simulink library "DAEMOT_Lib"  (R2019b)
settings: Solver=ode45  StartTime=0.0  StopTime=10.0  FixedStep=0.1  RelTol=1e-3
undefined symbols (not defined in the file or in its folder): Controller, CP, Ctrl, Ctrl_Fcn, Elec1, f, F2, Fluid, lag1, Mission, Moody, PropellerProp, rev_comms_sink
libraries: $bdroot x200, instrumentlib x21, simulink x5, dspsigops x2
(part 11 of 13)

== system DAEMOT_Lib/Electrical/Battery/Property ==
  I : Inport
  T_m : Inport  Port=2
  SOC : Inport  Port=3
  " " : Lookup  InputValues=cell.Ent_SOC  Table=cell.dUdt
  " " : Lookup  InputValues=cell.V_SOC  Table=cell.Vocv  LookUpMeth=Interpolation-Use End Values
  Fcn{1..5} (5 alike) : Fcn  Expr=((u(1)-u(3))/(1+exp(-50*u(2))))+u(3)
  Gain : Gain  Gain=Ns
  Mux : Mux  Inputs=7
  Mux{1..5} (5 alike) : Mux  Inputs=3
  n-D Lookup Table1 : Lookup_n-D  BreakpointsForDimension1=cell.RC_SOC_c  BreakpointsForDimension2=cell.Temp  BreakpointsForDimension3=[5, 7]  Table=cell.Rs_c  RndMeth=Simplest  InputSameDT=on
  n-D Lookup Table13 : Lookup_n-D  BreakpointsForDimension1=cell.RC_SOC_d  BreakpointsForDimension2=cell.Temp  BreakpointsForDimension3=[5, 7]  Table=cell.Rs_d  RndMeth=Simplest  InputSameDT=on
  n-D Lookup Table2 : Lookup_n-D  BreakpointsForDimension1=cell.RC_SOC_d  BreakpointsForDimension2=cell.Temp  BreakpointsForDimension3=[5, 7]  Table=cell.R1_d  RndMeth=Simplest  InputSameDT=on
  n-D Lookup Table3 : Lookup_n-D  BreakpointsForDimension1=cell.RC_SOC_c  BreakpointsForDimension2=cell.Temp  BreakpointsForDimension3=[5, 7]  Table=cell.R1_c  RndMeth=Simplest  InputSameDT=on
  n-D Lookup Table4 : Lookup_n-D  BreakpointsForDimension1=cell.RC_SOC_d  BreakpointsForDimension2=cell.Temp  BreakpointsForDimension3=[5, 7]  Table=cell.C1_d  RndMeth=Simplest  InputSameDT=on
  n-D Lookup Table5 : Lookup_n-D  BreakpointsForDimension1=cell.RC_SOC_c  BreakpointsForDimension2=cell.Temp  BreakpointsForDimension3=[5, 7]  Table=cell.C1_c  RndMeth=Simplest  InputSameDT=on
  n-D Lookup Table6 : Lookup_n-D  BreakpointsForDimension1=cell.RC_SOC_d  BreakpointsForDimension2=cell.Temp  BreakpointsForDimension3=[5, 7]  Table=cell.R2_d  RndMeth=Simplest  InputSameDT=on
  n-D Lookup Table7 : Lookup_n-D  BreakpointsForDimension1=cell.RC_SOC_c  BreakpointsForDimension2=cell.Temp  BreakpointsForDimension3=[5, 7]  Table=cell.R2_c  RndMeth=Simplest  InputSameDT=on
  n-D Lookup Table8 : Lookup_n-D  BreakpointsForDimension1=cell.RC_SOC_d  BreakpointsForDimension2=cell.Temp  BreakpointsForDimension3=[5, 7]  Table=cell.C2_d  RndMeth=Simplest  InputSameDT=on
  n-D Lookup Table9 : Lookup_n-D  BreakpointsForDimension1=cell.RC_SOC_c  BreakpointsForDimension2=cell.Temp  BreakpointsForDimension3=[5, 7]  Table=cell.C2_c  RndMeth=Simplest  InputSameDT=on
  Props : Outport
  wires:
  Gain/1 -> Mux/7
  Mux/1 -> Props/1
  " "/1 -> Gain/1  "V_ocv"
  " "/1 -> Mux/6  "dU_dt"
  Fcn1/1 -> Mux/1  "Rs"
  T_m/1 -> n-D Lookup Table9/2, n-D Lookup Table8/2, n-D Lookup Table7/2, n-D Lookup Table6/2, n-D Lookup Table5/2, n-D Lookup Table4/2, n-D Lookup Table3/2, n-D Lookup Table2/2, n-D Lookup Table1/2, n-D Lookup Table13/2
  SOC/1 -> n-D Lookup Table9/1, " "/1, " "/1, n-D Lookup Table8/1, n-D Lookup Table7/1, n-D Lookup Table6/1, n-D Lookup Table5/1, n-D Lookup Table4/1, n-D Lookup Table3/1, n-D Lookup Table2/1, n-D Lookup Table1/1, n-D Lookup Table13/1
  I/1 -> Mux2/2, Mux1/2, Mux5/2, Mux4/2, Mux3/2
  Fcn5/1 -> Mux/5  "C2"
  Fcn4/1 -> Mux/4  "R2"
  Fcn2/1 -> Mux/2  "R1"
  Fcn3/1 -> Mux/3  "C1"
  Mux2/1 -> Fcn1/1
  n-D Lookup Table1/1 -> Mux2/3
  n-D Lookup Table13/1 -> Mux2/1
  Mux1/1 -> Fcn2/1
  n-D Lookup Table2/1 -> Mux1/1
  n-D Lookup Table3/1 -> Mux1/3
  Mux3/1 -> Fcn3/1
  n-D Lookup Table4/1 -> Mux3/1
  n-D Lookup Table5/1 -> Mux3/3
  Mux4/1 -> Fcn4/1
  n-D Lookup Table6/1 -> Mux4/1
  n-D Lookup Table7/1 -> Mux4/3
  Mux5/1 -> Fcn5/1
  n-D Lookup Table8/1 -> Mux5/1
  n-D Lookup Table9/1 -> Mux5/3

== system DAEMOT_Lib/Electrical/Battery/Sink1 ==
  In1 : Inport
  tag scope: gdata_DAEMOT_LibElectricalBatterySink1=global
  wires:
  In1/1 -> [gdata_DAEMOT_LibElectricalBatterySink1]

== system DAEMOT_Lib/Electrical/Battery/Source1 ==
  Out1 : Outport
  wires:
  [NULL] -> Out1/1

== system DAEMOT_Lib/Electrical/Battery/Source2 ==
  Out1 : Outport
  wires:
  [NULL] -> Out1/1

== system DAEMOT_Lib/Electrical/Current Sink/Sink1 ==
  In1 : Inport
  tag scope: gdata_DAEMOT_LibElectricalCurrentSinkSink1=global
  wires:
  In1/1 -> [gdata_DAEMOT_LibElectricalCurrentSinkSink1]

== system DAEMOT_Lib/Electrical/Current Source/Source1 ==
  Out1 : Outport  VectorParamsAs1DForOutWhenUnconnected=off
  wires:
  [NULL] -> Out1/1

== system DAEMOT_Lib/Electrical/ESC/Data_Sink ==
  " " : Inport
  tag scope: gdata_ElectricalESCData_Sink=global
  wires:
  " "/1 -> [gdata_ElectricalESCData_Sink]

== system DAEMOT_Lib/Electrical/ESC/Sink1 ==
  In1 : Inport
  tag scope: gdata_DAEMOT_LibElectricalESCSink1=global
  wires:
  In1/1 -> [gdata_DAEMOT_LibElectricalESCSink1]

== system DAEMOT_Lib/Electrical/Effort Sink/Sink1 ==
  In1 : Inport
  tag scope: gdata_DAEMOT_LibElectricalEffortSinkSink1=global
  wires:
  In1/1 -> [gdata_DAEMOT_LibElectricalEffortSinkSink1]

== system DAEMOT_Lib/Electrical/Effort Source/Source1 ==
  Out1 : Outport  VectorParamsAs1DForOutWhenUnconnected=off
  wires:
  [NULL] -> Out1/1

== system DAEMOT_Lib/Electrical/Engine/Data_Sink ==
  " " : Inport
  tag scope: gdata_ElectricalEngineData_Sink=global
  wires:
  " "/1 -> [gdata_ElectricalEngineData_Sink]

== system DAEMOT_Lib/Electrical/Engine/Dynamic Saturation ==
  up : Inport
  u : Inport  Port=2
  dn : Inport  Port=3
  LowerRelop1 : RelationalOperator  DisableCoverage=on  Operator=>  OutDataTypeStr=boolean  ZeroCross=off  RndMeth=Nearest
  Switch : Switch  Criteria=u2 ~= 0  OutDataTypeStr=Inherit: Inherit via back propagation  ZeroCross=off
  Switch2 : Switch  Criteria=u2 ~= 0  OutMin=0  OutMax=1  OutDataTypeStr=Inherit: Inherit via back propagation  ZeroCross=off
  UpperRelop : RelationalOperator  DisableCoverage=on  Operator=<  OutDataTypeStr=boolean  ZeroCross=off  RndMeth=Nearest
  Out1 : Outport
  wires:
  Switch2/1 -> Out1/1
  up/1 -> Switch2/1, LowerRelop1/2
  UpperRelop/1 -> Switch/2
  dn/1 -> UpperRelop/2, Switch/1
  LowerRelop1/1 -> Switch2/2
  Switch/1 -> Switch2/3
  u/1 -> UpperRelop/1, Switch/3, LowerRelop1/1

== system DAEMOT_Lib/Electrical/Engine/Sink1 ==
  In1 : Inport
  tag scope: gdata_DAEMOT_LibElectricalEngineSink1=global
  wires:
  In1/1 -> [gdata_DAEMOT_LibElectricalEngineSink1]

== system DAEMOT_Lib/Electrical/Gearbox/Data_Sink ==
  " " : Inport
  tag scope: gdata_ElectricalGearboxData_Sink=global
  wires:
  " "/1 -> [gdata_ElectricalGearboxData_Sink]

== system DAEMOT_Lib/Electrical/Gearbox/Sink1 ==
  In1 : Inport
  tag scope: gdata_DAEMOT_LibElectricalGearboxSink1=global
  wires:
  In1/1 -> [gdata_DAEMOT_LibElectricalGearboxSink1]

== system DAEMOT_Lib/Electrical/Gearbox/Source1 ==
  Out1 : Outport
  wires:
  [NULL] -> Out1/1

== system DAEMOT_Lib/Electrical/Inverter/Data_Sink ==
  " " : Inport
  tag scope: gdata_ElectricalInverterData_Sink=global
  wires:
  " "/1 -> [gdata_ElectricalInverterData_Sink]

== system DAEMOT_Lib/Electrical/Inverter/Sink1 ==
  In1 : Inport
  tag scope: gdata_DAEMOT_LibElectricalInverterSink1=global
  wires:
  In1/1 -> [gdata_DAEMOT_LibElectricalInverterSink1]

== system DAEMOT_Lib/Electrical/Inverter/Source1 ==
  Out1 : Outport
  wires:
  [NULL] -> Out1/1

== system DAEMOT_Lib/Electrical/Inverter/Source2 ==
  Out1 : Outport
  wires:
  [NULL] -> Out1/1

== system DAEMOT_Lib/Electrical/Motor/Data_Sink ==
  " " : Inport
  tag scope: gdata_ElectricalMotorData_Sink=global
  wires:
  " "/1 -> [gdata_ElectricalMotorData_Sink]

== system DAEMOT_Lib/Electrical/Motor/Sink1 ==
  In1 : Inport
  tag scope: gdata_DAEMOT_LibElectricalMotorSink1=global
  wires:
  In1/1 -> [gdata_DAEMOT_LibElectricalMotorSink1]

== system DAEMOT_Lib/Electrical/Motor/Source1 ==
  Out1 : Outport
  wires:
  [NULL] -> Out1/1

== system DAEMOT_Lib/Electrical/Motor/Source2 ==
  Out1 : Outport
  wires:
  [NULL] -> Out1/1

== system DAEMOT_Lib/Electrical/MotorNoShaft/Data_Sink ==
  " " : Inport
  tag scope: gdata_ElectricalMotorNoShaftData_Sink=global
  wires:
  " "/1 -> [gdata_ElectricalMotorNoShaftData_Sink]

== system DAEMOT_Lib/Electrical/MotorNoShaft/Sink1 ==
  In1 : Inport
  tag scope: gdata_DAEMOT_LibElectricalMotorNoShaftSink1=global
  wires:
  In1/1 -> [gdata_DAEMOT_LibElectricalMotorNoShaftSink1]

== system DAEMOT_Lib/Electrical/MotorNoShaft/Source1 ==
  Out1 : Outport
  wires:
  [NULL] -> Out1/1

== system DAEMOT_Lib/Electrical/MotorNoShaft/Source2 ==
  Out1 : Outport
  wires:
  [NULL] -> Out1/1

== system DAEMOT_Lib/Electrical/Shaft/Data_Sink ==
  " " : Inport
  tag scope: gdata_ElectricalShaftData_Sink=global
  wires:
  " "/1 -> [gdata_ElectricalShaftData_Sink]

== system DAEMOT_Lib/Electrical/Shaft/Sink1 ==
  In1 : Inport
  tag scope: gdata_DAEMOT_LibElectricalShaftSink1=global
  wires:
  In1/1 -> [gdata_DAEMOT_LibElectricalShaftSink1]

== system DAEMOT_Lib/Electrical/Shaft/Source1 ==
  Out1 : Outport
  wires:
  [NULL] -> Out1/1

== system DAEMOT_Lib/Electrical/Speed Source/Source1 ==
  Out1 : Outport  VectorParamsAs1DForOutWhenUnconnected=off
  wires:
  [NULL] -> Out1/1

== system DAEMOT_Lib/Electrical/Torque Sink/Sink1 ==
  In1 : Inport
  tag scope: gdata_DAEMOT_LibElectricalTorqueSinkSink1=global
  wires:
  In1/1 -> [gdata_DAEMOT_LibElectricalTorqueSinkSink1]

== system DAEMOT_Lib/Electrical/UAV/Property ==
  v : Inport
  w : Inport  Port=2
  " C_L" : Lookup  InputValues=PropellerProp.J  Table=PropellerProp.C_L
  " C_T" : Lookup  InputValues=PropellerProp.J  Table=PropellerProp.C_T
  " eta" : Lookup  InputValues=PropellerProp.J  Table=PropellerProp.eta
  Divide : Product  Inputs=*/
  Gain : Gain  Gain=2*pi
  Gain1 : Gain  Gain=d
  Mux : Mux
  Scope : Scope
  Props : Outport  VectorParamsAs1DForOutWhenUnconnected=off
  wires:
  Mux/1 -> Props/1
  w/1 -> Gain1/1
  v/1 -> Gain/1
  Gain/1 -> Divide/1
  Gain1/1 -> Divide/2
  Divide/1 -> " eta"/1, " C_L"/1, " C_T"/1, Scope/1, Mux/1  "J"
  " C_T"/1 -> Mux/2  "C_T"
  " C_L"/1 -> Mux/3  "C_L"
  " eta"/1 -> Mux/4  "eta"

== system DAEMOT_Lib/Electrical/Ultracapacitor/Props ==
  Constant : Constant  Value=R_i
  Constant1 : Constant  Value=C_i0
  Constant2 : Constant  Value=C_i1
  Constant3 : Constant  Value=R_d
  Constant4 : Constant  Value=C_d
  Constant5 : Constant  Value=R_l
  Constant6 : Constant  Value=C_l
  Constant7 : Constant  Value=R_leak
  Mux : Mux  Inputs=8
  props : Outport  VectorParamsAs1DForOutWhenUnconnected=off
  wires:
  Constant/1 -> Mux/1
  Constant1/1 -> Mux/2
  Mux/1 -> props/1
  Constant2/1 -> Mux/3
  Constant3/1 -> Mux/4
  Constant4/1 -> Mux/5
  Constant5/1 -> Mux/6
  Constant6/1 -> Mux/7
  Constant7/1 -> Mux/8

== system DAEMOT_Lib/Electrical/Ultracapacitor/Sink1 ==
  In1 : Inport
  Scope : Scope
  tag scope: gdata_DAEMOT_LibElectricalUltracapacitorSink1=global
  wires:
  In1/1 -> Scope/1, [gdata_DAEMOT_LibElectricalUltracapacitorSink1]

== system DAEMOT_Lib/Electrical/Voltage Sink/Sink1 ==
  In1 : Inport
  tag scope: gdata_DAEMOT_LibElectricalVoltageSinkSink1=global
  wires:
  In1/1 -> [gdata_DAEMOT_LibElectricalVoltageSinkSink1]

== system DAEMOT_Lib/Electrical/Voltage Source/Source1 ==
  Out1 : Outport  VectorParamsAs1DForOutWhenUnconnected=off
  wires:
  [NULL] -> Out1/1

== system DAEMOT_Lib/Electrical/wye2del/Data_Sink ==
  " " : Inport
  tag scope: gdata_Electricalwye2delData_Sink=global
  wires:
  " "/1 -> [gdata_Electricalwye2delData_Sink]

== system DAEMOT_Lib/Electrical/wye2del/Sink1 ==
  In1 : Inport
  tag scope: gdata_DAEMOT_LibElectricalwye2delSink1=global
  wires:
  In1/1 -> [gdata_DAEMOT_LibElectricalwye2delSink1]

== system DAEMOT_Lib/Electrical/wye2del/Source1 ==
  Out1 : Outport
  wires:
  [NULL] -> Out1/1

== system DAEMOT_Lib/Legacy Components/Fan1/Sink1 ==
  In1 : Inport
  tag scope: gdata_DAEMOT_LibLegacyComponentsFan1Sink1=global
  wires:
  In1/1 -> [gdata_DAEMOT_LibLegacyComponentsFan1Sink1]

== system DAEMOT_Lib/Legacy Components/Flow Flow Source (Pressure)/Source1 ==
  Out1 : Outport  VectorParamsAs1DForOutWhenUnconnected=off
  wires:
  [gdata_Thermal_System_BUSM2FSink2] -> Out1/1

== system DAEMOT_Lib/Legacy Components/Flow Source (Mass Flow Rate)/Source1 ==
  Out1 : Outport  VectorParamsAs1DForOutWhenUnconnected=off
  wires:
  [gdata_Thermal_System_BUSM2FSink2] -> Out1/1

== system DAEMOT_Lib/Legacy Components/Flow Split_Junction_Wall/Source1 ==
  Out1 : Outport  VectorParamsAs1DForOutWhenUnconnected=off
  wires:
  [NULL] -> Out1/1

== system DAEMOT_Lib/Legacy Components/Graph Sink/Sink1 ==
  In1 : Inport
  tag scope: gdata_DAEMOT_LibLegacyComponentsGraphSinkSink1=global
  wires:
  In1/1 -> [gdata_DAEMOT_LibLegacyComponentsGraphSinkSink1]

== system DAEMOT_Lib/Legacy Components/Graph Source/Source1 ==
  Out1 : Outport  VectorParamsAs1DForOutWhenUnconnected=off
  wires:
  [NULL] -> Out1/1

== system DAEMOT_Lib/Legacy Components/Heat Sink (Temp)/Sink1 ==
  In1 : Inport
  tag scope: gdata_DAEMOT_LibLegacyComponentsHeatSinkTempSink1=global
  wires:
  In1/1 -> [gdata_DAEMOT_LibLegacyComponentsHeatSinkTempSink1]

== system DAEMOT_Lib/Legacy Components/Pipe_M_to_M/Props ==
  P : Inport
  T : Inport  Port=2
  Divide : Product  Inputs=*/
  Fcn : Fcn  Expr=0.99*u
  Subtract : Sum  Inputs=+-
  Subtract1 : Sum  Inputs=+-
  n-D Lookup Table1 : Lookup_n-D  BreakpointsForDimension1=Fluid.P  BreakpointsForDimension2=Fluid.T  BreakpointsForDimension3=[5, 7]  Table=Fluid.Rho_pt  ExtrapMethod=Clip  UseLastTableValue=on  RndMeth=Simplest  InputSameDT=on
  n-D Lookup Table5 : Lookup_n-D  BreakpointsForDimension1=Fluid.P  BreakpointsForDimension2=Fluid.T  BreakpointsForDimension3=[5, 7]  Table=Fluid.Rho_pt  ExtrapMethod=Clip  UseLastTableValue=on  RndMeth=Simplest  InputSameDT=on
  Rho : Outport  VectorParamsAs1DForOutWhenUnconnected=off
  dRho_dP : Outport  Port=2  VectorParamsAs1DForOutWhenUnconnected=off
  wires:
  T/1 -> n-D Lookup Table5/2, n-D Lookup Table1/2
  n-D Lookup Table5/1 -> Subtract/1, Rho/1
  P/1 -> Subtract1/1, Fcn/1, n-D Lookup Table5/1
  Fcn/1 -> n-D Lookup Table1/1, Subtract1/2
  n-D Lookup Table1/1 -> Subtract/2
  Subtract/1 -> Divide/1
  Subtract1/1 -> Divide/2
  Divide/1 -> dRho_dP/1

== system DAEMOT_Lib/Legacy Components/Power Sink (Current)/Sink1 ==
  In1 : Inport
  tag scope: gdata_DAEMOT_LibLegacyComponentsPowerSinkCurrentSink1=global
  wires:
  In1/1 -> [gdata_DAEMOT_LibLegacyComponentsPowerSinkCurrentSink1]

== system DAEMOT_Lib/Legacy Components/Power Source (Voltage)/Source1 ==
  Out1 : Outport  VectorParamsAs1DForOutWhenUnconnected=off
  wires:
  [NULL] -> Out1/1

== system DAEMOT_Lib/Legacy Components/Static Flow Split/Sink1 ==
  In1 : Inport
  tag scope: gdata_DAEMOT_LibLegacyComponentsStaticFlowSplitSink1=global
  wires:
  In1/1 -> [gdata_DAEMOT_LibLegacyComponentsStaticFlowSplitSink1]

== system DAEMOT_Lib/Legacy Components/Static Flow Split/Source1 ==
  Out1 : Outport  VectorParamsAs1DForOutWhenUnconnected=off
  wires:
  [gdata_Thermal_System_BUSFuelPumSink1] -> Out1/1

== system DAEMOT_Lib/Legacy Components/UDP_Controller_SR_old/From Controller ==
  MEASUREMENTS1 : Subsystem  mask{n_meas=out_size}
      mask prompts: n_meas "Number of measurements from LabView"
      mask init:
      | h = gcbh;
      | param = get(h);
      | blk = [param.Path, '/', param.Name,'/UDP Receive'];
      | h = get_param(blk,'handle');
      | 
      | set_param(h,'DataSize',['[',num2str(n_meas),' 1]'])
      mask Display:
      | if n_meas > 1
      |     port_label('output',1,['Mux - ',num2str(n_meas),' signals'])
      | else
      |     port_label('output',1,['Mux - ',num2str(n_meas),' signal'])
      | end
  Out1 : Outport  VectorParamsAs1DForOutWhenUnconnected=off
  wires:
  MEASUREMENTS1/1(Out) -> Out1/1

== system DAEMOT_Lib/Legacy Components/UDP_Controller_SR_old/To Controller ==
  " " : Inport
  UDP Send : instrumentlib/UDP Send  Host=localhost  Port=61176  LocalPort=61177  EnablePortSharing=off  ByteOrder=BigEndian  OutputDatagramPacketSize=512  EnableBlockingMode=on  LocalAddress=0.0.0.0
      settings: SourceProductName=Instrument Control Toolbox
  wires:
  " "/1 -> UDP Send/1

== system DAEMOT_Lib/Legacy Components/UDP_Controller_old/From Controller ==
  " " : Inport
  UDP Send : instrumentlib/UDP Send  Host=localhost  Port=61167  LocalPort=61166  EnablePortSharing=off  ByteOrder=BigEndian  OutputDatagramPacketSize=512  EnableBlockingMode=on  LocalAddress=0.0.0.0
      settings: SourceProductName=Instrument Control Toolbox
  Zero-Order Hold : ZeroOrderHold  Commented=through  SampleTime=0.1
  wires:
  " "/1 -> Zero-Order Hold/1
  Zero-Order Hold/1 -> UDP Send/1

== system DAEMOT_Lib/Legacy Components/UDP_Controller_old/To Controller ==
  UDP Receive : instrumentlib/UDP Receive  Host=localhost  Port=61177  LocalPort=61176  EnablePortSharing=off  GetLatestData=off  DataSize=[1 1]  DataType=double  ASCIIFormatting=%f,  Terminator=LF  ByteOrder=BigEndian  EnableBlockingMode=on  Timeout=6  SampleTime=1  LocalAddress=0.0.0.0
      settings: SourceProductName=Instrument Control Toolbox
  Out : Outport  VectorParamsAs1DForOutWhenUnconnected=off
  wires:
  UDP Receive/1 -> Out/1

== system DAEMOT_Lib/Legacy Components/Upper to Lower Edge Preview_old/Mission Preview1 ==
  Trajectory : Inport
  Time : Inport  Port=2
  Add : Sum
  Bias : Bias  Bias=+dt_l*linspace(0,(hor_l-1),hor_l)
  Constant : Constant  Value=0:dt_l:((hor_u)*dt_u-1)  VectorParams1D=off
  Digital Clock : DigitalClock  SampleTime=dt_l
  Display{,1..3} (4 alike) : Display
  Lookup Table Dynamic : simulink/Lookup Tables/Lookup Table Dynamic  LookUpMeth=Use Input Below  OutDataType=fixdt('double')  OutScaling=[]  OutputDataTypeScalingMode=Specify via dialog  OutDataTypeStr=double  DoSatur=off
      settings: SourceProductName=Simulink
  MATLAB Function : MATLAB Function  Commented=on  TreatAsAtomicUnit=on
  MATLAB Function1 : MATLAB Function  TreatAsAtomicUnit=on
  Reshape : Reshape  OutputDimensionality=Row vector (2-D)
  Reshape1 : Reshape
  References : Outport  VectorParamsAs1DForOutWhenUnconnected=off
  wires:
  Reshape/1 -> References/1, Display3/1
  MATLAB Function1/1(y) -> Lookup Table Dynamic/3, Display2/1
  Reshape1/1 -> MATLAB Function1/1(u)
  Constant/1 -> Add/2
  Time/1 -> Add/1
  Add/1 -> Lookup Table Dynamic/2, Display1/1
  Trajectory/1 -> Reshape1/1
  Lookup Table Dynamic/1 -> Reshape/1
  Bias/1 -> Lookup Table Dynamic/1, Display/1
  Digital Clock/1 -> Bias/1

== system DAEMOT_Lib/Support Functions/Generic Graph Model/Variant Subsystem ==
  Inputs : Inport
  Source Vertex : Inport  Port=2
  Source Edge : Inport  Port=3
  DAE Graph : Subsystem  VariantControl=DAE_Graph
  Dynamic Graph : Subsystem  VariantControl=Dynamic_Graph
  States : Outport
  Power Flows : Outport  Port=2

== system DAEMOT_Lib/Support Functions/Generic Sink/Sink1 ==
  In1 : Inport
  tag scope: gdata_DAEMOT_LibSupportFunctionsGenericSinkSink1=global
  wires:
  In1/1 -> [gdata_DAEMOT_LibSupportFunctionsGenericSinkSink1]

== system DAEMOT_Lib/Support Functions/Generic Source/Source1 ==
  Out1 : Outport  VectorParamsAs1DForOutWhenUnconnected=off
  wires:
  [NULL] -> Out1/1

== system DAEMOT_Lib/Support Functions/Real-Time Communication/LabVIEW_UDP ==
  " " : Inport
  Bus Creator : BusCreator  Inputs=15
  Bus Selector : BusSelector  OutputSignals=SimulinkTime,MCM_EnablePropESC,MCM_RPMCommand,MCM_EnableBattCharge,MCM_EnableSGESC,MCM_EnableICE,MCM_GenIMax,MCM_BattIMax,Dyno_Enable,Dyno_C0,Dyno_C1,Dyno_C2,DCDC_Enable0,DCDC_Enable1,DCDC_Enable2,DCDC_Voltage0,DCDC_Voltage1,DCDC_Voltage2,DCDC_Current0,DCDC_Current1,DCDC_Current2,ELoad_voltage_limit_enabled,ELoad_voltage_limit  OutputAsBus=on
  Bus to Vector : BusToVector
  Check_NaN1 : Subsystem  mask{N=n_in}
      mask prompts: N "Number of Signals"
  Demux : Demux  Outputs=15
  UDP Receive : instrumentlib/UDP Receive  Host=localhost  Port=61556  LocalPort=61557  EnablePortSharing=off  GetLatestData=off  DataSize=[15 1]  DataType=double  ASCIIFormatting=%f,  Terminator=LF  ByteOrder=BigEndian  EnableBlockingMode=on  Timeout=10  SampleTime=0.1  LocalAddress=0.0.0.0
      settings: SourceProductName=Instrument Control Toolbox
  UDP Send : instrumentlib/UDP Send  Host=localhost  Port=61556  LocalPort=61557  EnablePortSharing=off  ByteOrder=BigEndian  OutputDatagramPacketSize=512  EnableBlockingMode=on  LocalAddress=0.0.0.0
      settings: SourceProductName=Instrument Control Toolbox
  Zero-Order Hold : ZeroOrderHold  SampleTime=0.1
  Out : Outport  VectorParamsAs1DForOutWhenUnconnected=off
  wires:
  Bus to Vector/1 -> Zero-Order Hold/1
  Bus Selector/1 -> Bus to Vector/1
  Zero-Order Hold/1 -> UDP Send/1
  " "/1 -> Bus Selector/1
  Bus Creator/1 -> Out/1
  UDP Receive/1 -> Check_NaN1/1(In1)
  Check_NaN1/1(Out1) -> Demux/1
  Demux/1 -> Bus Creator/1  "Test Time"
  Demux/2 -> Bus Creator/2  "PackVoltage"
  Demux/3 -> Bus Creator/3  "(MCM) Bus Voltage [V]"
  Demux/4 -> Bus Creator/4  "(DCDC) Bus Voltage [V]"
  Demux/5 -> Bus Creator/5  "Shunt_SystemBatt"
  Demux/6 -> Bus Creator/6  "(MCM) Bus DC Current [A]"
  Demux/7 -> Bus Creator/7  "Shunt_VoltageSteps"
  Demux/8 -> Bus Creator/8  "(DCDC) Bus DC Current [A]"
  Demux/9 -> Bus Creator/9  "(MCM) Prop DC Current [A]"
  Demux/10 -> Bus Creator/10  "(MCM) Prop Speed [RPM]"
  Demux/11 -> Bus Creator/11  "(MCM) SG DC Current [A]"
  Demux/12 -> Bus Creator/12  "ELoad_voltage_measured"
  Demux/13 -> Bus Creator/13  "ELoad_current_measured"
  Demux/14 -> Bus Creator/14  "Shunt_Channel_A_Load"
  Demux/15 -> Bus Creator/15  "(DCDC) Duty Cycle A"

== system DAEMOT_Lib/Support Functions/Real-Time Communication/UDP_Controller ==
  note: the zero order hold should be unnecessary
      | because everything here has a Ctrl.dt update
      | rate. When operating with Parallel simulations,
      | this block will start in sync with the main simulation.
      | Once the controller calls, the main and parallel sims
      | will operate asynchronously. Upon controller call completion,
      | data is immediately sent to the main sim. The main sim will receive
      | that data at it's update rate (likely 10Hz). At this point, the main sim
      | is ahead of the parallel sim by the time it took to call
      | the controller rounded up to the nearest .1s (assuming
      | 10Hz). However, the parallel sim can now immediately forward
      | simulate to the next UDP recieve and wait for data (The
      | parallel sim is ahead of the main sim for this period). Once the
      | main sim catches up in time, data is sent to and recieved by the
      | parallel sim and the process repeats.
  Controller : Subsystem  TreatAsAtomicUnit=on  SystemSampleTime=0.1
  Display : Display
  Display1 : Display
  From Controller : Subsystem  Priority=3  TreatAsAtomicUnit=on  SystemSampleTime=0.1
  Reshape1 : Reshape  OutputDimensionality=Column vector (2-D)
  Scope : Scope
  Scope1 : Scope
  UDP Receive : instrumentlib/UDP Receive  Priority=2  Host=localhost  Port=61177  LocalPort=61176  EnablePortSharing=off  GetLatestData=off  DataSize=[10 1]  DataType=double  ASCIIFormatting=%f,  Terminator=LF  ByteOrder=BigEndian  EnableBlockingMode=on  Timeout=5.1  SampleTime=0.1  LocalAddress=0.0.0.0
      settings: SourceProductName=Instrument Control Toolbox
  Zero-Order Hold : ZeroOrderHold  Commented=through  SampleTime=Ctrl.dt
  wires:
  Reshape1/1 -> Controller/1(In1), Scope/1
  UDP Receive/1 -> Reshape1/1
  Controller/1(Out1) -> Display/1, Zero-Order Hold/1
  Zero-Order Hold/1 -> Display1/1, From Controller/1(" "), Scope1/1

== system DAEMOT_Lib/Support Functions/Real-Time Communication/UDP_Controller_Debug ==
  Controller : MATLABFcn  MATLABFcn=Controller(u)  OutputDimensions=10
  From Controller : Subsystem  Priority=3  TreatAsAtomicUnit=on  SystemSampleTime=0.1
  Reshape1 : Reshape  OutputDimensionality=Column vector (2-D)
  Scope : Scope
  Scope1 : Scope
  UDP Receive : instrumentlib/UDP Receive  Priority=2  Host=localhost  Port=61177  LocalPort=61176  EnablePortSharing=off  GetLatestData=off  DataSize=[10 1]  DataType=double  ASCIIFormatting=%f,  Terminator=LF  ByteOrder=BigEndian  EnableBlockingMode=on  Timeout=5.1  SampleTime=0.1  LocalAddress=0.0.0.0
      settings: SourceProductName=Instrument Control Toolbox
  wires:
  Controller/1 -> From Controller/1(" "), Scope1/1
  Reshape1/1 -> Scope/1, Controller/1
  UDP Receive/1 -> Reshape1/1

== system DAEMOT_Lib/Support Functions/Real-Time Communication/UDP_Controller_Recieve ==
  Bus Creator : BusCreator  Inputs=2
  From Controller : Subsystem  Commented=on  TreatAsAtomicUnit=on  SystemSampleTime=.1
  Reshape : Reshape
  Sample and Hold : dspsigops/Sample and Hold  trig=Rising edge  initCond=Initial  latchinput=off
  TCP/IP Receive : instrumentlib/TCP//IP Receive  Priority=2  Commented=on  Host=localhost  Port=50000  DataSize=[1 1]  EnableBlockingMode=on  Timeout=3  SampleTime=.1  DataType=double  ByteOrder=BigEndian  ASCIIFormatting=%f,  Terminator=LF
      settings: SourceProductName=Instrument Control Toolbox
  UDP Receive : instrumentlib/UDP Receive  Priority=3  Host=localhost  Port=61166  LocalPort=61167  EnablePortSharing=off  GetLatestData=off  DataSize=[10 1]  DataType=double  ASCIIFormatting=%f,  Terminator=LF  ByteOrder=BigEndian  EnableBlockingMode=off  Timeout=10  SampleTime=0.1  LocalAddress=0.0.0.0
      settings: SourceProductName=Instrument Control Toolbox
  Zero-Order Hold : ZeroOrderHold  SampleTime=0.1
  Output : Outport  VectorParamsAs1DForOutWhenUnconnected=off
  wires:
  Bus Creator/1 -> Output/1
  Zero-Order Hold/1 -> Bus Creator/2  "Output at Update"
  Sample and Hold/1 -> Zero-Order Hold/1, Bus Creator/1  "Immediate Output"
  UDP Receive/2 -> Sample and Hold/Trigger
  UDP Receive/1 -> Reshape/1  "Recieved"
  Reshape/1 -> Sample and Hold/1

== system DAEMOT_Lib/Support Functions/Real-Time Communication/UDP_Controller_Recieve_Debug ==
  Reshape : Reshape
  Scope : Scope
  UDP Receive : instrumentlib/UDP Receive  Priority=3  Host=localhost  Port=61166  LocalPort=61167  EnablePortSharing=off  GetLatestData=off  DataSize=[10 1]  DataType=double  ASCIIFormatting=%f,  Terminator=LF  ByteOrder=BigEndian  EnableBlockingMode=on  Timeout=10  SampleTime=0.1  LocalAddress=0.0.0.0
      settings: SourceProductName=Instrument Control Toolbox
  Controller Output : Outport  VectorParamsAs1DForOutWhenUnconnected=off
  wires:
  Reshape/1 -> Controller Output/1, Scope/1
  UDP Receive/1 -> Reshape/1  "Recieved"

== system DAEMOT_Lib/Support Functions/Real-Time Communication/UDP_Controller_Send ==
  Controller Input : Inport
  Reshape11 : Reshape  OutputDimensionality=Column vector (2-D)
  To Controller : Subsystem  Priority=1  TreatAsAtomicUnit=on  SystemSampleTime=0.1
  wires:
  Reshape11/1 -> To Controller/1(In1)
  Controller Input/1 -> Reshape11/1

== system DAEMOT_Lib/Support Functions/Real-Time Communication/UDP_Controller_Send_Debug ==
  Controller Input : Inport
  Reshape11 : Reshape  OutputDimensionality=Column vector (2-D)
  To Controller : Subsystem  Priority=1  TreatAsAtomicUnit=on  SystemSampleTime=0.1
  wires:
  Controller Input/1 -> Reshape11/1
  Reshape11/1 -> To Controller/1(In1)

== system DAEMOT_Lib/Support Functions/Upper to Lower Edge Preview/Mission Preview1 ==
  Trajectory : Inport
  Time : Inport  Port=2
  Add : Sum
  Bias : Bias  Bias=+dt_l*linspace(0,(hor_l-1),hor_l)
  Constant : Constant  Value=0:dt_l:((hor_u)*dt_u-dt_l)  VectorParams1D=off
  Digital Clock : DigitalClock  SampleTime=dt_l
  Interpreted MATLAB Function : MATLABFcn  MATLABFcn=repmat(u,1,dt_u/dt_l)  Output1D=off
  Lookup Table Dynamic : simulink/Lookup Tables/Lookup Table Dynamic  LookUpMeth=Use Input Below  OutDataType=fixdt('double')  OutScaling=[]  OutputDataTypeScalingMode=Specify via dialog  OutDataTypeStr=fixdt('double')  DoSatur=off
      settings: SourceProductName=Simulink
  Math Function : Math  Operator=transpose  SaturateOnIntegerOverflow=on
  Reshape : Reshape  OutputDimensionality=Row vector (2-D)
  Reshape1 : Reshape  OutputDimensionality=Column vector (2-D)
  Reshape2 : Reshape  OutputDimensionality=Column vector (2-D)
  Reshape3 : Reshape  OutputDimensionality=Column vector (2-D)
  References : Outport
  wires:
  Reshape1/1 -> Lookup Table Dynamic/2
  Math Function/1 -> Reshape3/1
  Reshape2/1 -> Interpreted MATLAB Function/1
  Interpreted MATLAB Function/1 -> Math Function/1
  Trajectory/1 -> Reshape2/1
  Reshape/1 -> References/1
  Reshape3/1 -> Lookup Table Dynamic/3
  Constant/1 -> Add/2
  Time/1 -> Add/1
  Add/1 -> Reshape1/1
  Lookup Table Dynamic/1 -> Reshape/1
  Bias/1 -> Lookup Table Dynamic/1
  Digital Clock/1 -> Bias/1

== system DAEMOT_Lib/Thermal/Flow Split_Junction/Source1 ==
  Out1 : Outport  VectorParamsAs1DForOutWhenUnconnected=off
  wires:
  [NULL] -> Out1/1

== system DAEMOT_Lib/Thermal/PCM Module/Props ==
  Constant1 : Constant  Value=k_l
  Constant10 : Constant  Value=rho_h
  Constant12 : Constant  Value=rho_f
  Constant13 : Constant  Value=k_f
  Constant14 : Constant  Value=c_f
  Constant2 : Constant  Value=T_melt
  Constant3 : Constant  Value=L_pcm
  Constant4 : Constant  Value=rho_pcm
  Constant5 : Constant  Value=c_pcm
  Constant6 : Constant  Value=beta
  Constant7 : Constant  Value=nu
  Constant8 : Constant  Value=c_h
  Constant9 : Constant  Value=k_h
  Vector Concatenate : Concatenate  NumInputs=13
  props : Outport  VectorParamsAs1DForOutWhenUnconnected=off
  wires:
  Constant14/1 -> Vector Concatenate/11
  Constant13/1 -> Vector Concatenate/12
  Constant12/1 -> Vector Concatenate/13
  Constant10/1 -> Vector Concatenate/10
  Constant9/1 -> Vector Concatenate/9
  Constant8/1 -> Vector Concatenate/8
  Vector Concatenate/1 -> props/1
  Constant7/1 -> Vector Concatenate/7
  Constant6/1 -> Vector Concatenate/6
  Constant5/1 -> Vector Concatenate/5
  Constant4/1 -> Vector Concatenate/4
  Constant3/1 -> Vector Concatenate/3
  Constant2/1 -> Vector Concatenate/2
  Constant1/1 -> Vector Concatenate/1

== system DAEMOT_Lib/Legacy Components/UDP_Controller_SR_old/From Controller/MEASUREMENTS1 ==
  Terminator : Terminator
  UDP Receive : instrumentlib/UDP Receive  Host=localhost  Port=61166  LocalPort=61167  EnablePortSharing=off  GetLatestData=off  DataSize=[1 1]  DataType=double  ASCIIFormatting=%f,  Terminator=LF  ByteOrder=BigEndian  EnableBlockingMode=off  Timeout=5  SampleTime=0.1  LocalAddress=0.0.0.0
      settings: SourceProductName=Instrument Control Toolbox
  Out : Outport  VectorParamsAs1DForOutWhenUnconnected=off
  wires:
  UDP Receive/1 -> Out/1
  UDP Receive/2 -> Terminator/1

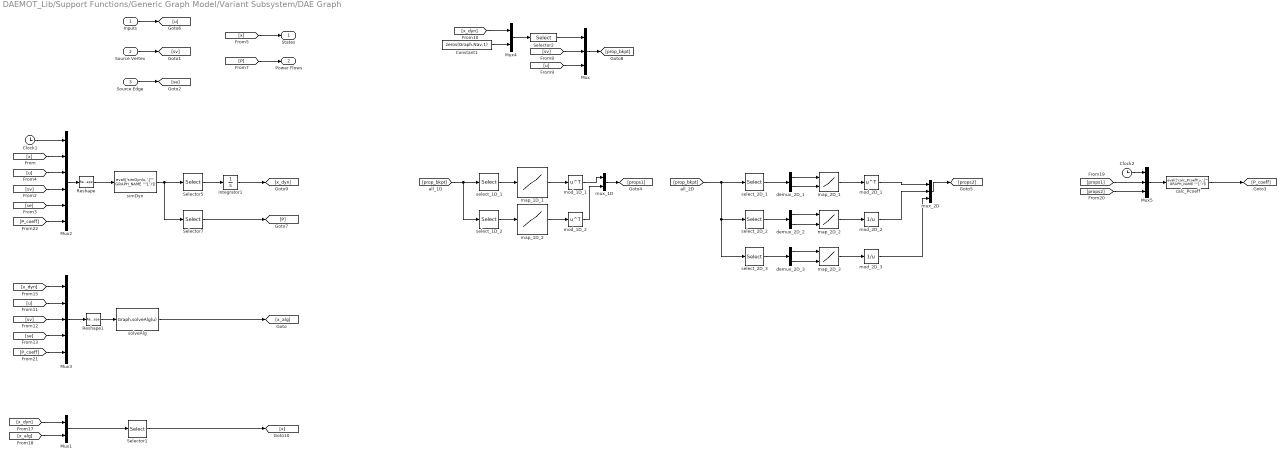
== system DAEMOT_Lib/Support Functions/Generic Graph Model/Variant Subsystem/DAE Graph ==
  Inputs : Inport
  Source Vertex : Inport  Port=2
  Source Edge : Inport  Port=3
  Clock1 : Clock
  Clock2 : Clock
  Constant1 : Constant  Value=zeros(Graph.Nav,1)
  Integrator1 : Integrator  InitialCondition=Graph.x_int(Graph.Caps(1:Graph.Nv) ~= 0)
  Mux : Mux  Inputs=3
  Mux1 : Mux  Inputs=2
  Mux2 : Mux  Inputs=6
  Mux3 : Mux  Inputs=5
  Mux4 : Mux  Inputs=2
  Mux5 : Mux  Inputs=3
  Reshape : Reshape  OutputDimensionality=Column vector (2-D)
  Reshape1 : Reshape  OutputDimensionality=Row vector (2-D)
  Selector1 : Selector  InputPortWidth=Graph.Nv  IndexOptions=Index vector (dialog)  Indices=Graph.dyn_alg2x  OutputSizes=1
  Selector2 : Selector  InputPortWidth=Graph.Nv  IndexOptions=Index vector (dialog)  Indices=Graph.dyn_alg2x  OutputSizes=1
  Selector5 : Selector  InputPortWidth=Graph.Ndv+Graph.Ne*Graph.Nd  IndexOptions=Index vector (dialog)  Indices=1:Graph.Ndv  OutputSizes=1
  Selector7 : Selector  InputPortWidth=Graph.Ndv+Graph.Ne*Graph.Nd  IndexOptions=Index vector (dialog)  Indices=[Graph.Ndv+1:Graph.Ndv+Graph.Ne*Graph.Nd]  OutputSizes=1
  calc_Pcoeff : MATLABFcn  MATLABFcn=eval(['calc_Pcoeff(u,',['''' GRAPH_NAME ''''],')'])  OutputDimensions=Graph.Ne*Graph.Nd
  demux_2D_1 : Demux  Outputs=2
  demux_2D_2 : Demux  Outputs=2
  demux_2D_3 : Demux  Outputs=2
  map_1D_1 : Lookup_n-D  NumberOfTableDimensions=1  BreakpointsForDimension1=Elec1.Props.D1_map{3,1}  Table=Elec1.Props.D1_map{4,1}  InternalRulePriority=Speed  RndMeth=Simplest  InputSameDT=on
  map_1D_2 : Lookup_n-D  NumberOfTableDimensions=1  BreakpointsForDimension1=Elec1.Props.D1_map{3,2}  Table=Elec1.Props.D1_map{4,2}  InternalRulePriority=Speed  RndMeth=Simplest  InputSameDT=on
  map_2D_1 : Lookup_n-D  BreakpointsForDimension1=Elec1.Props.D2_map{3,1}{1,1}  BreakpointsForDimension2=Elec1.Props.D2_map{3,1}{2,1}  Table=Elec1.Props.D2_map{4,1}'  InternalRulePriority=Speed  RndMeth=Simplest  InputSameDT=on
  map_2D_2 : Lookup_n-D  BreakpointsForDimension1=Elec1.Props.D2_map{3,2}{1,1}  BreakpointsForDimension2=Elec1.Props.D2_map{3,2}{2,1}  Table=Elec1.Props.D2_map{4,2}'  InternalRulePriority=Speed  RndMeth=Simplest  InputSameDT=on
  map_2D_3 : Lookup_n-D  BreakpointsForDimension1=Elec1.Props.D2_map{3,3}{1,1}  BreakpointsForDimension2=Elec1.Props.D2_map{3,3}{2,1}  Table=Elec1.Props.D2_map{4,3}'  InternalRulePriority=Speed  RndMeth=Simplest  InputSameDT=on
  mod_1D_1 : Math  Operator=transpose  SignedPower=off  SaturateOnIntegerOverflow=on
  mod_1D_2 : Math  Operator=transpose  SignedPower=off  SaturateOnIntegerOverflow=on
  mod_2D_1 : Math  Operator=transpose  SignedPower=off  SaturateOnIntegerOverflow=on
  mod_2D_2 : Math  Operator=reciprocal  SignedPower=off  SaturateOnIntegerOverflow=on
  mod_2D_3 : Math  Operator=reciprocal  SignedPower=off  SaturateOnIntegerOverflow=on
  mux_1D : Mux  Inputs=2
  mux_2D : Mux  Inputs=3
  select_1D_1 : Selector  InputPortWidth=Elec1.Nv+10+7  IndexOptions=Index vector (dialog)  Indices=Elec1.Props.D1_map{1,1}  OutputSizes=1
  select_1D_2 : Selector  InputPortWidth=Elec1.Nv+10+7  IndexOptions=Index vector (dialog)  Indices=Elec1.Props.D1_map{1,2}  OutputSizes=1
  select_2D_1 : Selector  InputPortWidth=Elec1.Nv+10+7  IndexOptions=Index vector (dialog)  Indices=Elec1.Props.D2_map{1,1}  OutputSizes=1
  select_2D_2 : Selector  InputPortWidth=Elec1.Nv+10+7  IndexOptions=Index vector (dialog)  Indices=Elec1.Props.D2_map{1,2}  OutputSizes=1
  select_2D_3 : Selector  InputPortWidth=Elec1.Nv+10+7  IndexOptions=Index vector (dialog)  Indices=Elec1.Props.D2_map{1,3}  OutputSizes=1
  simDyn : MATLABFcn  MATLABFcn=eval(['simDyn(u,',['''' GRAPH_NAME ''''],')'])  OutputDimensions=Graph.Ndv+Graph.Ne*Graph.Nd
  solveAlg : MATLABFcn  MATLABFcn=Graph.solveAlg(u)  OutputDimensions=Graph.Nav
  States : Outport
  Power Flows : Outport  Port=2
  wires:
  Mux/1 -> [prop_bkpt]
  [u] -> Mux/3
  [sv] -> Mux/2
  Inputs/1 -> [u]
  Source Edge/1 -> [se]
  Source Vertex/1 -> [sv]
  [x] -> States/1
  [P] -> Power Flows/1
  mux_2D/1 -> [props2]
  mux_1D/1 -> [props1]
  Mux2/1 -> Reshape/1
  Selector5/1 -> Integrator1/1
  Clock1/1 -> Mux2/1
  Selector7/1 -> [P]
  simDyn/1 -> Selector5/1, Selector7/1
  [x] -> Mux2/2
  Reshape/1 -> simDyn/1
  [u] -> Mux2/3
  [sv] -> Mux2/4
  [se] -> Mux2/5
  [u] -> Mux3/2
  [sv] -> Mux3/3
  [se] -> Mux3/4
  Mux3/1 -> Reshape1/1
  solveAlg/1 -> [x_alg]
  [x_dyn] -> Mux3/1
  Reshape1/1 -> solveAlg/1
  [prop_bkpt] -> select_1D_1/1, select_1D_2/1
  select_1D_1/1 -> map_1D_1/1
  map_1D_1/1 -> mod_1D_1/1
  mod_1D_1/1 -> mux_1D/1
  [prop_bkpt] -> select_2D_2/1, select_2D_3/1, select_2D_1/1
  select_2D_1/1 -> demux_2D_1/1
  demux_2D_1/1 -> map_2D_1/1
  demux_2D_1/2 -> map_2D_1/2
  map_2D_1/1 -> mod_2D_1/1
  mod_2D_1/1 -> mux_2D/1
  select_2D_2/1 -> demux_2D_2/1
  demux_2D_2/1 -> map_2D_2/1
  demux_2D_2/2 -> map_2D_2/2
  map_2D_2/1 -> mod_2D_2/1
  mod_2D_2/1 -> mux_2D/2
  select_2D_3/1 -> demux_2D_3/1
  demux_2D_3/1 -> map_2D_3/1
  demux_2D_3/2 -> map_2D_3/2
  map_2D_3/1 -> mod_2D_3/1
  mod_2D_3/1 -> mux_2D/3
  [x_dyn] -> Mux1/1
  [x_alg] -> Mux1/2
  Mux1/1 -> Selector1/1
  Selector1/1 -> [x]
  Selector2/1 -> Mux/1
  Mux4/1 -> Selector2/1
  [x_dyn] -> Mux4/1
  Constant1/1 -> Mux4/2
  Mux5/1 -> calc_Pcoeff/1
  [props1] -> Mux5/2
  [props2] -> Mux5/3
  Clock2/1 -> Mux5/1
  calc_Pcoeff/1 -> [P_coeff]
  [P_coeff] -> Mux3/5
  [P_coeff] -> Mux2/6
  Integrator1/1 -> [x_dyn]
  select_1D_2/1 -> map_1D_2/1
  map_1D_2/1 -> mod_1D_2/1
  mod_1D_2/1 -> mux_1D/2

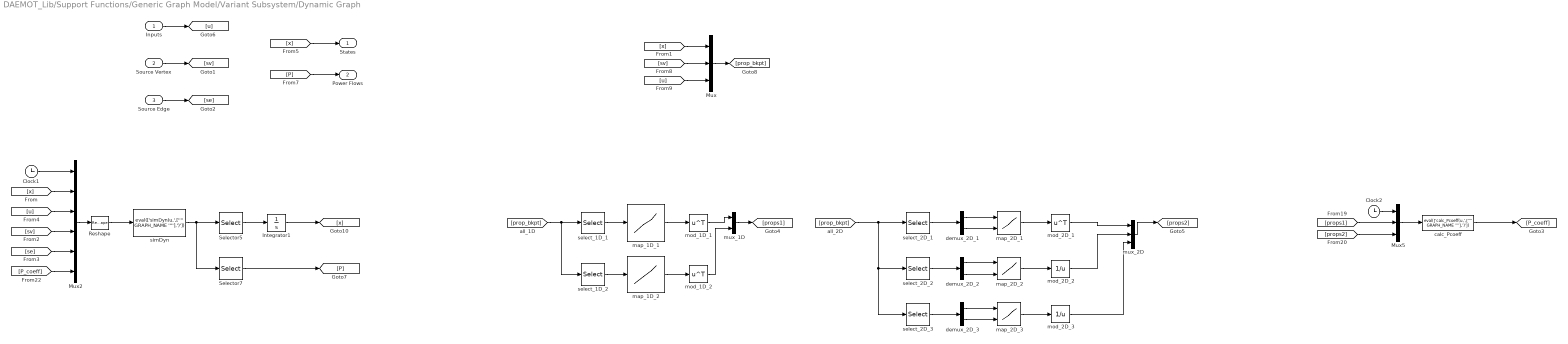
== system DAEMOT_Lib/Support Functions/Generic Graph Model/Variant Subsystem/Dynamic Graph ==
  Inputs : Inport
  Source Vertex : Inport  Port=2
  Source Edge : Inport  Port=3
  Clock1 : Clock
  Clock2 : Clock
  Integrator1 : Integrator  InitialCondition=Graph.x_int(Graph.Caps(1:Graph.Nv) ~= 0)
  Mux : Mux  Inputs=3
  Mux2 : Mux  Inputs=6
  Mux5 : Mux  Inputs=3
  Reshape : Reshape  OutputDimensionality=Column vector (2-D)
  Selector5 : Selector  InputPortWidth=Graph.Ndv+Graph.Ne*Graph.Nd  IndexOptions=Index vector (dialog)  Indices=1:Graph.Ndv  OutputSizes=1
  Selector7 : Selector  InputPortWidth=Graph.Ndv+Graph.Ne*Graph.Nd  IndexOptions=Index vector (dialog)  Indices=[Graph.Ndv+1:Graph.Ndv+Graph.Ne*Graph.Nd]  OutputSizes=1
  calc_Pcoeff : MATLABFcn  MATLABFcn=eval(['calc_Pcoeff(u,',['''' GRAPH_NAME ''''],')'])  OutputDimensions=Graph.Ne*Graph.Nd
  demux_2D_1 : Demux  Outputs=2
  demux_2D_2 : Demux  Outputs=2
  demux_2D_3 : Demux  Outputs=2
  map_1D_1 : Lookup_n-D  NumberOfTableDimensions=1  BreakpointsForDimension1=Elec1.Props.D1_map{3,1}  Table=Elec1.Props.D1_map{4,1}  InternalRulePriority=Speed  RndMeth=Simplest  InputSameDT=on
  map_1D_2 : Lookup_n-D  NumberOfTableDimensions=1  BreakpointsForDimension1=Elec1.Props.D1_map{3,2}  Table=Elec1.Props.D1_map{4,2}  InternalRulePriority=Speed  RndMeth=Simplest  InputSameDT=on
  map_2D_1 : Lookup_n-D  BreakpointsForDimension1=Elec1.Props.D2_map{3,1}{1,1}  BreakpointsForDimension2=Elec1.Props.D2_map{3,1}{2,1}  Table=Elec1.Props.D2_map{4,1}'  InternalRulePriority=Speed  RndMeth=Simplest  InputSameDT=on
  map_2D_2 : Lookup_n-D  BreakpointsForDimension1=Elec1.Props.D2_map{3,2}{1,1}  BreakpointsForDimension2=Elec1.Props.D2_map{3,2}{2,1}  Table=Elec1.Props.D2_map{4,2}'  InternalRulePriority=Speed  RndMeth=Simplest  InputSameDT=on
  map_2D_3 : Lookup_n-D  BreakpointsForDimension1=Elec1.Props.D2_map{3,3}{1,1}  BreakpointsForDimension2=Elec1.Props.D2_map{3,3}{2,1}  Table=Elec1.Props.D2_map{4,3}'  InternalRulePriority=Speed  RndMeth=Simplest  InputSameDT=on
  mod_1D_1 : Math  Operator=transpose  SignedPower=off  SaturateOnIntegerOverflow=on
  mod_1D_2 : Math  Operator=transpose  SignedPower=off  SaturateOnIntegerOverflow=on
  mod_2D_1 : Math  Operator=transpose  SignedPower=off  SaturateOnIntegerOverflow=on
  mod_2D_2 : Math  Operator=reciprocal  SignedPower=off  SaturateOnIntegerOverflow=on
  mod_2D_3 : Math  Operator=reciprocal  SignedPower=off  SaturateOnIntegerOverflow=on
  mux_1D : Mux  Inputs=2
  mux_2D : Mux  Inputs=3
  select_1D_1 : Selector  InputPortWidth=Elec1.Nv+10+7  IndexOptions=Index vector (dialog)  Indices=Elec1.Props.D1_map{1,1}  OutputSizes=1
  select_1D_2 : Selector  InputPortWidth=Elec1.Nv+10+7  IndexOptions=Index vector (dialog)  Indices=Elec1.Props.D1_map{1,2}  OutputSizes=1
  select_2D_1 : Selector  InputPortWidth=Elec1.Nv+10+7  IndexOptions=Index vector (dialog)  Indices=Elec1.Props.D2_map{1,1}  OutputSizes=1
  select_2D_2 : Selector  InputPortWidth=Elec1.Nv+10+7  IndexOptions=Index vector (dialog)  Indices=Elec1.Props.D2_map{1,2}  OutputSizes=1
  select_2D_3 : Selector  InputPortWidth=Elec1.Nv+10+7  IndexOptions=Index vector (dialog)  Indices=Elec1.Props.D2_map{1,3}  OutputSizes=1
  simDyn : MATLABFcn  MATLABFcn=eval(['simDyn(u,',['''' GRAPH_NAME ''''],')'])  OutputDimensions=Graph.Ndv+Graph.Ne*Graph.Nd
  States : Outport
  Power Flows : Outport  Port=2
  wires:
  mod_2D_3/1 -> mux_2D/3
  demux_2D_2/1 -> map_2D_2/1
  [x] -> Mux/1
  select_2D_3/1 -> demux_2D_3/1
  simDyn/1 -> Selector5/1, Selector7/1
  mod_2D_1/1 -> mux_2D/1
  demux_2D_1/1 -> map_2D_1/1
  mux_1D/1 -> [props1]
  mod_2D_2/1 -> mux_2D/2
  map_1D_1/1 -> mod_1D_1/1
  [prop_bkpt] -> select_1D_1/1, select_1D_2/1
  [prop_bkpt] -> select_2D_2/1, select_2D_3/1, select_2D_1/1
  demux_2D_3/2 -> map_2D_3/2
  map_2D_2/1 -> mod_2D_2/1
  [x] -> States/1
  demux_2D_2/2 -> map_2D_2/2
  select_2D_1/1 -> demux_2D_1/1
  [u] -> Mux2/3
  Mux2/1 -> Reshape/1
  select_1D_1/1 -> map_1D_1/1
  Selector7/1 -> [P]
  [se] -> Mux2/5
  [sv] -> Mux2/4
  Reshape/1 -> simDyn/1
  [P] -> Power Flows/1
  mod_1D_1/1 -> mux_1D/1
  mux_2D/1 -> [props2]
  Inputs/1 -> [u]
  Source Vertex/1 -> [sv]
  Clock1/1 -> Mux2/1
  Selector5/1 -> Integrator1/1
  [u] -> Mux/3
  Source Edge/1 -> [se]
  Clock2/1 -> Mux5/1
  demux_2D_3/1 -> map_2D_3/1
  Mux/1 -> [prop_bkpt]
  [sv] -> Mux/2
  [props1] -> Mux5/2
  [props2] -> Mux5/3
  select_2D_2/1 -> demux_2D_2/1
  map_2D_1/1 -> mod_2D_1/1
  [x] -> Mux2/2
  Mux5/1 -> calc_Pcoeff/1
  demux_2D_1/2 -> map_2D_1/2
  map_2D_3/1 -> mod_2D_3/1
  Integrator1/1 -> [x]
  [P_coeff] -> Mux2/6
  calc_Pcoeff/1 -> [P_coeff]
  select_1D_2/1 -> map_1D_2/1
  map_1D_2/1 -> mod_1D_2/1
  mod_1D_2/1 -> mux_1D/2

== system DAEMOT_Lib/Support Functions/Real-Time Communication/LabVIEW_UDP/Check_NaN1 ==
  In1 : Inport
  Bias1 : Bias  Bias=1:N
  Data Type Conversion2 : DataTypeConversion  OutDataTypeStr=double
  Gain2 : Gain  Gain=N
  IsNaN2 : RelationalOperator  Operator=isNaN  OutDataTypeStr=boolean  RndMeth=Simplest
  Memory3 : Memory  InitialCondition=zeros(1,N)  InheritSampleTime=on
  Mux1 : Mux  Inputs=2
  Selector1 : Selector  InputPortWidth=2*N  IndexOptions=Index vector (port)  Indices=[1 3]  OutputSizes=1
  Out1 : Outport
  wires:
  [old] -> Mux1/2
  Bias1/1 -> Selector1/2
  In1/1 -> Mux1/1, IsNaN2/1
  IsNaN2/1 -> Data Type Conversion2/1
  Gain2/1 -> Bias1/1
  Selector1/1 -> Out1/1, Memory3/1
  Data Type Conversion2/1 -> Gain2/1
  Mux1/1 -> Selector1/1
  Memory3/1 -> [old]

== system DAEMOT_Lib/Support Functions/Real-Time Communication/UDP_Controller/Controller ==
  In1 : Inport
  Constant : Constant  Commented=on  Value=lag1
  Controller : MATLABFcn  MATLABFcn=[1*u(1)]  OutputDimensions=10
  Controller1 : MATLABFcn  Commented=on  MATLABFcn=consumeTime  OutputDimensions=1
  Display : Display  Commented=on
  Out1 : Outport
  wires:
  Constant/1 -> Controller1/1
  In1/1 -> Controller/1
  Controller1/1 -> Display/1
  Controller/1 -> Out1/1

== system DAEMOT_Lib/Support Functions/Real-Time Communication/UDP_Controller/From Controller ==
  " " : Inport
  UDP Send : instrumentlib/UDP Send  Priority=3  Host=localhost  Port=61167  LocalPort=61166  EnablePortSharing=off  ByteOrder=BigEndian  OutputDatagramPacketSize=512  EnableBlockingMode=on  LocalAddress=0.0.0.0
      settings: SourceProductName=Instrument Control Toolbox
  wires:
  " "/1 -> UDP Send/1

== system DAEMOT_Lib/Support Functions/Real-Time Communication/UDP_Controller_Debug/From Controller ==
  " " : Inport
  Mux : Mux  Inputs=2
  Scope1 : Scope
  Scope2 : Scope
  Selector1 : Selector  IndexOptions=Index vector (dialog)  Indices=1  OutputSizes=1
  UDP Send : instrumentlib/UDP Send  Priority=3  Host=localhost  Port=61167  LocalPort=61166  EnablePortSharing=off  ByteOrder=BigEndian  OutputDatagramPacketSize=512  EnableBlockingMode=on  LocalAddress=0.0.0.0
      settings: SourceProductName=Instrument Control Toolbox
  wires:
  Mux/1 -> Scope2/1
  Selector1/1 -> Scope1/1
  " "/1 -> Mux/1, Mux/2, UDP Send/1, Selector1/1

== system DAEMOT_Lib/Support Functions/Real-Time Communication/UDP_Controller_Recieve/From Controller ==
  MEASUREMENTS1 : Subsystem  mask{n_meas=out_size}
      mask prompts: n_meas "Number of measurements from LabView"
      mask init:
      | h = gcbh;
      | param = get(h);
      | blk = [param.Path, '/', param.Name,'/UDP Receive'];
      | h = get_param(blk,'handle');
      | 
      | set_param(h,'DataSize',['[',num2str(n_meas),' 1]'])
      mask Display:
      | if n_meas > 1
      |     port_label('output',1,['Mux - ',num2str(n_meas),' signals'])
      | else
      |     port_label('output',1,['Mux - ',num2str(n_meas),' signal'])
      | end
  Scope1 : Scope
  Selector1 : Selector  IndexOptions=Index vector (dialog)  Indices=1  OutputSizes=1
  Out1 : Outport  VectorParamsAs1DForOutWhenUnconnected=off
  wires:
  MEASUREMENTS1/1(Out) -> Selector1/1, Out1/1
  Selector1/1 -> Scope1/1

== system DAEMOT_Lib/Support Functions/Real-Time Communication/UDP_Controller_Send/To Controller ==
  In1 : Inport
  UDP Send : instrumentlib/UDP Send  Priority=2  Host=localhost  Port=61176  LocalPort=61177  EnablePortSharing=off  ByteOrder=BigEndian  OutputDatagramPacketSize=512  EnableBlockingMode=on  LocalAddress=0.0.0.0
      settings: SourceProductName=Instrument Control Toolbox
  wires:
  In1/1 -> UDP Send/1

== system DAEMOT_Lib/Support Functions/Real-Time Communication/UDP_Controller_Send_Debug/To Controller ==
  In1 : Inport
  UDP Send : instrumentlib/UDP Send  Priority=2  Host=localhost  Port=61176  LocalPort=61177  EnablePortSharing=off  ByteOrder=BigEndian  OutputDatagramPacketSize=512  EnableBlockingMode=on  LocalAddress=0.0.0.0
      settings: SourceProductName=Instrument Control Toolbox
  wires:
  In1/1 -> UDP Send/1

== system DAEMOT_Lib/Support Functions/Real-Time Communication/UDP_Controller_Recieve/From Controller/MEASUREMENTS1 ==
  Scope : Scope  Commented=on
  TCP/IP Receive : instrumentlib/TCP//IP Receive  Commented=on  Host=localhost  Port=50000  DataSize=[1 1]  EnableBlockingMode=on  Timeout=10  SampleTime=.1  DataType=double  ByteOrder=BigEndian  ASCIIFormatting=%f,  Terminator=LF
      settings: SourceProductName=Instrument Control Toolbox
  UDP Receive : instrumentlib/UDP Receive  Priority=3  Commented=on  Host=localhost  Port=61166  LocalPort=61167  EnablePortSharing=off  GetLatestData=off  DataSize=[1 1]  DataType=double  ASCIIFormatting=%f,  Terminator=LF  ByteOrder=BigEndian  EnableBlockingMode=off  Timeout=33  SampleTime=.1  LocalAddress=0.0.0.0
      settings: SourceProductName=Instrument Control Toolbox
  Out : Outport  VectorParamsAs1DForOutWhenUnconnected=off
  wires:
  TCP/IP Receive/1 -> Out/1
  UDP Receive/2 -> Scope/1

== matlab function DAEMOT_Lib/Thermal/Flow Split_Junction/Dynamic_Flow_Split_Junction ==
  data: x input; Mdot_in input; Mdot_out input; T_in input; x_dot output; D parameter; L parameter; t parameter; E parameter; v parameter; rho input; E_fluid input
function x_dot  = Dynamic_Flow_Split_Junction(x,Mdot_in,Mdot_out,T_in,D,L,t,E,v,rho,E_fluid)

% Constants and Conversions
Mdot_in_tot     = sum(Mdot_in);     % Total mass flow rate in
Mdot_out_tot    = sum(Mdot_out);    % Total mass flow rate out
V               = pi*D^2/4*L;       % Volume

% Parse states
T      = x(1);                  % Temperature of the tank
P      = x(2);                  % Pressure at bottom of the tank

% Calculate state derivatives
T_dot = (dot(Mdot_in,T_in)-sum(Mdot_out)*T)/(rho*V);  % Split/Junc temperature
P_dot = (Mdot_in_tot-Mdot_out_tot)/(V*rho*(1/E_fluid+D*(1-v/2)/(t*E))); % Split/Junc pressure

% Mux state derivatives
x_dot  = [T_dot,P_dot];

end
